simulink model "LADRC1"  (R2023a)
settings: Solver=VariableStepAuto  StartTime=0.0  StopTime=20  RelTol=1e-3
settings Model: Creator=belov  LastModifiedBy=belov

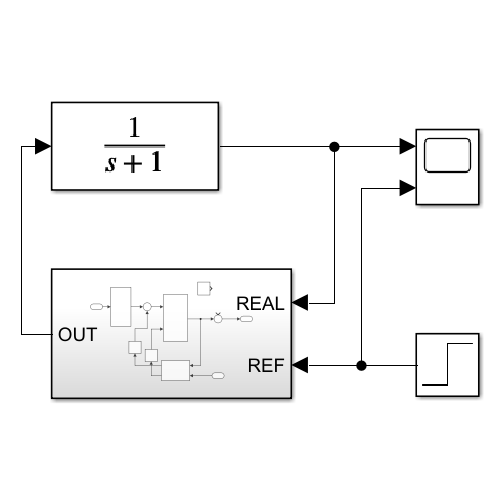
[thumbnail: Simulink's stored preview of the top-level diagram]
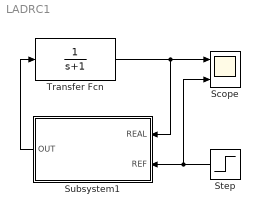
== system LADRC1 ==
  Scope : Scope  NumInputPorts=2
  Step : Step  SampleTime=0
  Subsystem1 : Subsystem
  Transfer Fcn : TransferFcn  Denominator=[1 1]
  wires:
  Transfer Fcn/1 -> Subsystem1/1(REAL), Scope/1
  Step/1 -> Subsystem1/2(REF), Scope/2
  Subsystem1/1(OUT) -> Transfer Fcn/1

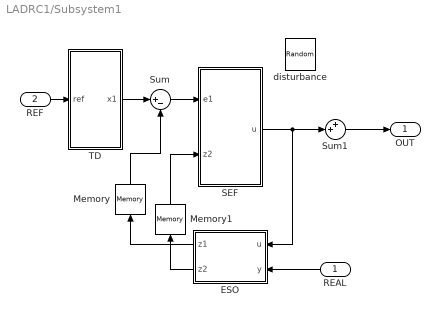
== system LADRC1/Subsystem1 ==
  REAL : Inport
  REF : Inport  Port=2
  ESO : MATLAB Function  TreatAsAtomicUnit=on  SystemSampleTime=0.001
  Memory : Memory
  Memory1 : Memory
  SEF : MATLAB Function  TreatAsAtomicUnit=on  SystemSampleTime=0.001
  Sum : Sum  Inputs=|+-
  Sum1 : Sum  Inputs=++|
  TD : MATLAB Function  TreatAsAtomicUnit=on  SystemSampleTime=0.001
  disturbance : UniformRandomNumber  Minimum=-0.1  Maximum=0.1  SampleTime=0.1
  OUT : Outport
  wires:
  ESO/1(z1) -> Memory/1
  REF/1 -> TD/1(ref)
  TD/1(x1) -> Sum/1
  Memory/1 -> Sum/2
  ESO/2(z2) -> Memory1/1
  Memory1/1 -> SEF/2(z2)
  Sum/1 -> SEF/1(e1)
  SEF/1(u) -> Sum1/2, ESO/1(u)
  REAL/1 -> ESO/2(y)
  Sum1/1 -> OUT/1

== matlab function LADRC1/Subsystem1/SEF ==
  data: e1 input; u output; z2 input
function u = SEF(e1, z2)

b0 = 1;

wc = 1;

a1 = wc;

u0 = a1 * e1;
u = (u0 - z2) / b0;
% u = 1 / b0 * (a1 * e1 + a2 * e2 + a3 * e3 + z4);

end

== matlab function LADRC1/Subsystem1/TD ==
  data: ref input; x1 output
function x1 = TD(ref)

persistent x1_;

h = 0.001; % 步长
r = 10;

if isempty(x1_)
    x1_=0;
end


x1 = x1_ + h * (-r * x1_ + r * ref);

x1_ = x1;

end

== matlab function LADRC1/Subsystem1/ESO ==
  data: u input; z1 output; y input; z2 output
function [z1, z2] = ESO(u, y)

wo = 5;
b0 = 1;

beta1 = 2 * wo;
beta2 = wo * wo;

h = 0.001;

persistent z1_ z2_;

if isempty(z1_)
    z1_ = 0;
end
if isempty(z2_)
    z2_ = 0;
end

z1 = z1_ + h * (-beta1 * z1_ + z2_ + b0 * u + beta1 * y);
z2 = z2_ + h * (-beta2 * z1_ + beta2 * y);

z1_ = z1;
z2_ = z2;
end
